simulink model "BattEv_Simscape"  (R2023b)
settings: Solver=ode23t  StartTime=0  StopTime=inf  RelTol=1e-3  EnableMultiTasking=on
model workspace (MAT data in the model file):
  Active_Scenario_Index = 1
  BattCurrent = [0 0.1 0.2 0.3 0.4 0.5 0.6 0.7 0.8 0.9 1 1.1 ... (49482 elements, 24741x2)]
  BattSocInit = 0.75
  BattTempInit = 25
  Battery.SOC_LUT = [0.01 0.02 0.03 0.04 0.05 0.06 0.07 0.08 0.09 0.1 0.11 0.12 0.13 0.14 0.15 0.16 0.17 0.18 0.19 0.2 0.21 0.22 0.23 0.24 0.25 0.26 0.27 0.28 0.29 0.3 0.31 0.32 0.33 0.34 0.35 0.36 0.37 0.38 0.39 0.4 0.41 0.42 0.43 0.44 0.45 0.46 0.47 0.48 0.49 0.5 0.51 0.52 0.53 0.54 0.55 0.56 0.57 0.58 0.59 0.6 0.61 0.62 0.63 0.64 0.65 0.66 0.67 0.68 0.69 0.7 0.71 0.72 0.73 0.74 0.75 0.76 0.77 0.78 0.79 0.8 0.81 0.82 0.83 0.84 0.85 0.86 0.87 0.88 0.89 0.9 0.91 0.92 0.93 0.94 0.95 0.96 0.97 0.98 0.99 1]
  Battery.Temperature_LUT = [-10 0 25 40]
  Battery.Capacity_LUT = [4.04528301887 4.19622641509 4.8 4.73962264151]
  Battery.Em_LUT = [2.67308083891 2.74411674384 2.80408613071 2.86247711994 2.90851059763 2.94904306488 2.9829846776 3.01467102589 3.04031502638 3.06256828113 3.08180972392 3.09994219643 ... (400 elements, 100x4)]
  Battery.R0_LUT = [0.0569026752707 0.0575506938969 0.0576730924021 0.0575627404981 0.0573787336615 0.0571931123197 0.0568199985482 0.056411926464 0.0561974340667 0.0560805640861 0.0557640899305 0.055275807865 ... (400 elements, 100x4)]
  Battery.R1_LUT = [0.0035 0.0035 0.0035 0.0035 0.0035 0.0035 0.0035 0.0035 0.0035 0.0035 0.0035 0.0035 ... (400 elements, 100x4)]
  Battery.C1_LUT = [5000 5000 5000 5000 5000 5000 5000 5000 5000 5000 5000 5000 ... (400 elements, 100x4)]
  Battery.Mass = 0.047
  Battery.ThermalMass = 44
  Battery.R_bleed = 20
  Battery.h_conv = 5
  Battery.cell_area = 0.0037
  Battery.TempInit = 25
  Battery.SOCInit = 0.75
  Battery.Model = 'panasonic ncr18650bd'
  Battery.DischargeCycle_LUT = [1 5 9 13 17 21 25 29 33 37 41 45 49 53 57 61 65 69 73 77 81 85 89 93 97 101 105 109 113 117 121 125 129 133 137 141 145 149 153 157 161 165 169 173 177 181 185 189 193 197 201 205 209 213 217 221 225 229 233 237 241 245 249 253 257 261 265 269 273 277 281 285 289 293 297 301 305 309 313 317]
  Battery.deltaEm_LUT = [0 -0.363115641304 -0.600096647258 -0.689070000839 -0.76773380251 -0.846397604181 -0.926368385458 -0.992711297521 -1.05704974111 -1.12227693902 -1.19018070587 -1.25808447272 -1.31699459748 -1.35876443799 -1.40168267642 -1.44460091485 -1.48751915327 -1.5304373917 -1.57335563013 -1.62198241593 -1.67232184498 -1.71858340023 -1.76179802551 -1.8050126508 -1.84822727608 -1.8917937136 -1.93575272784 -1.97971174208 -2.02367075632 -2.06762977056 -2.11171979109 -2.15588700406 -2.19980020032 -2.24365853098 -2.28751686164 -2.33137519231 -2.37523352297 -2.41909185363 -2.45982559031 -2.49599372373 -2.53216185715 -2.56832999058 -2.604498124 -2.64066625743 -2.67683439085 -2.71300252428 -2.7491706577 -2.78367585394 -2.81632179346 -2.8483348579 -2.88034792233 -2.91236098677 -2.94437405121 -2.97638711564 -3.00840018008 -3.04041324451 -3.07260346059 -3.10359008254 -3.13082308991 -3.15805609728 -3.18528910464 -3.21252211201 -3.23975511938 -3.26698812675 -3.29422113412 -3.32122400938 -3.3463475604 -3.37152613073 -3.39670470105 -3.42188327138 -3.4470618417 -3.47224041203 -3.49938358795 -3.52900276724 -3.55862194653 -3.58824112582 -3.6178603051 -3.64748858268 -3.67711690909 -3.70674523549]
  Battery.deltaCapacity_LUT = [0 -0.860019120059 -1.71332421702 -2.0819400264 -2.45055583577 -2.81917164515 -3.18778745452 -3.48884924257 -3.7808148236 -4.07278040463 -4.36474598566 -4.6567115667 -4.91000721732 -5.08494410056 -5.2598809838 -5.43481786703 -5.60975475027 -5.78469163351 -5.95962851674 -6.13456539998 -6.30950228322 -6.47026795816 -6.62044510558 -6.77062225299 -6.92079940041 -7.07097654783 -7.22115369524 -7.37133084266 -7.52150799007 -7.67168513749 -7.82230984162 -7.97319825819 -8.12408667477 -8.27497509134 -8.42586350792 -8.57675192449 -8.72764034107 -8.87852875764 -9.01789522921 -9.13717923376 -9.25646323831 -9.37574724285 -9.4950312474 -9.61431525195 -9.73359925649 -9.85288326104 -9.97216726558 -10.0914512701 -10.2059878191 -10.3183039593 -10.4306200996 -10.5429362398 -10.65525238 -10.7675685203 -10.8798846605 -10.9922008008 -11.104516941 -11.2125891929 -11.3075699376 -11.4025506823 -11.4975314271 -11.5925121718 -11.6874929166 -11.7824736613 -11.877454406 -11.9716325175 -12.0588579537 -12.1460833899 -12.2333088261 -12.3205342623 -12.4077596986 -12.4949851348 -12.5890165008 -12.6916254178 -12.7942343349 -12.8968432519 -12.999452169 -13.102061086 -13.2046700031 -13.3072789201]
  Battery.cond_thickness = 0.001
  Battery.thermal_conductivity = 205
  CellType = 1
  EV_current = 200
  EV_motion = [20 4 0.8]
  EV_sf = 2000
  Fs = 0
  Fv = 0.0025
  Jcomp = 0.0227
  Ki = 251.3274
  Kisa = 346.6583
  Kp_d = 0.47149
  Kp_q = 0.52125
  Ksa = 85.4316
  Ksf = 1996.2651
  Ld = 0.0003752
  Ldq = [0.0003752 0.0004148]
  Lq = 0.0004148
  Mechanical = [0.0227 0.0025 0]
  Np_Module = 31
  Ns_Module = 24
  NumModules = 4
  OverCellVoltageLimit = 4.19999980927
  P = 4
  PolePairs = 4
  R_bleed = 20
  Rs = 0.2
  T_eff_bp = [0 32.1428571429 64.2857142857 96.4285714286 128.571428571 160.714285714 192.857142857 225 257.142857143 289.285714286 321.428571429 353.571428571 385.714285714 417.857142857 450]
  T_env = 30
  T_init = 303.15
  T_max = 450
  T_mtpa = [0 13.3131834767 26.6278836885 39.9456159322 53.2678926341 66.5962219318 79.9321062746 93.277041051 106.632513247 120.000000141]
  T_set = 20.5
  Tc = 0.02
  TempInit = 288.15
  TestCase = 1
  UnderCellVoltageLimit = 2.5
  ba = 3.4029
  cell_area = 0.101908
  efficiency_table = [86.7  86.7  86.7  86.7  86.7  86.7  86.7  86.7  86.7  86.7  86.7  86.7  86.7  86.7  86.7; 86.7  86.7  86.7  86.7  86.7  86.7  86.7  86.7  86.7  86.7  86.7  86.7  86.7  86.7  86.7; 86.7  86.7  91.8  91.8  91.8  91.8  91.8  91.8  91.8  91.8  89.76  89.76  89.76  89.76  89.76; 86.7  86.7  93.84  93.84  93.84  93.84  93.84  93.84  93.84  93.84  93.84  91.8  91.8  91.8  91.8; 86.7  86.7  93.84  93.84  94.86  94.86  94.86  94.86  93.84  93.84  93.84  91.8  91.8  91.8  91.8; 86.7  86.7  94.86  95.88  95.88  95.88  95.88  95.88  95.88  95.88  95.88  95.88  95.88  95.88  95.88; 86.7  86.7  94.86  95.88  95.88  96.9  96.9  96.9  96.9  96.9  96.9  96.9  96.9  96.9  96.9; 86.7  86.7  94.86  95.88  95.88  96.9  96.9  96.9  96.9  96.9  96.9  96.9  96.9  96.9  96.9; 86.7  86.7  94.86  95.88  96.9  96.9  96.9  96.9  96.9  96.9  96.9  96.9  96.9  96.9  96.9; 86.7  86.7  94.86  95.88  96.9  96.9  96.9  96.9  96.9  96.9  96.9  96.9  96.9  96.9  96.9; 86.7  86.7  94.86  95.88  95.88  95.88  95.88  95.88  95.88  95.88  95.88  95.88  95.88  95.88  95.88; 86.7  86.7  91.8  93.84  94.86  94.86  94.86  94.86  94.86  94.86  94.86  94.86  94.86  94.86  94.86]
  h_conv = 5
  id_mtpa = [0 -0.114523352646 -0.457989076459 -1.03008464374 -1.83029075221 -2.85788367342 -4.11193850568 -5.59133329791 -7.29475400168 -9.22070020138]
  idq0 = [0 0]
  idq_limits = [-9.220699542 166.993501392 167.247872355]
  iq_mtpa = [0 18.5827440345 37.1633719111 55.7397734896 74.3098506185 92.871523015 111.422734008 129.961456105 148.485696337 166.993501356]
  lambda_pm = 0.1194
  losses_table = [0  0  0  0  0  0  0  0  0  0  0  0  0  0  0; 0  0  0  0  0  0  0  0  0  0  0  0  0  0  0; 0  0  0  0  0  0  0  0  0  0  0  0  0  0  0; 0  0  0  0  0  0  0  0  0  0  0  0  0  0  0; 0  0  0  0  0  0  0  0  0  0  0  0  0  0  0; 0  0  0  0  0  0  0  0  0  0  0  0  0  0  0; 0  0  0  0  0  0  0  0  0  0  0  0  0  0  0; 0  0  0  0  0  0  0  0  0  0  0  0  0  0  0; 0  0  0  0  0  0  0  0  0  0  0  0  0  0  0; 0  0  0  0  0  0  0  0  0  0  0  0  0  0  0; 0  0  0  0  0  0  0  0  0  0  0  0  0  0  0; 0  0  0  0  0  0  0  0  0  0  0  0  0  0  0]
  mdot_rev = 0.01
  mechanical = [0.0227 0.0025 0]
  omega_init = 0
  pipe.length = 75
  pipe.Dh = 2.5
  pipe.area = 4.90873852123
  power_max = 211000
  pump.omega = 4000
  pump.displacement = 40
  radiator.area_air = 0.15
  radiator.volume_air = 0.01
  radiator.area_liquid = 0.000314159265359
  radiator.volume_liquid = 0.000157079632679
  radiator.mdot_air = [0.1 8]
  radiator.mdot_liquid = [0.1 5]
  radiator.SD = [1  9; 2  10]
  radiator.dp_air = [0.003 0.01]
  radiator.dp_liquid = [0.005 0.02]
  t_sim = 2474
  tank.volume = 10
  tank.area = 0.0625
  tank.area_wall = 0.375
  theta_init = 0
  torque_max = 450
  ts = 0.1
  valve.area = 4.90873852123
  valve.opening = 4.81056375081
  valve.area_leak = 1e-05
  w_eff_bp = [0 1600 3200 4477.56 4800 6400 8000 9600 11200 12800 14400 16000]
libraries: autolibpowerinfoutils x10, fl_lib x7, nesl_utility_internal x6, ee_lib x1
(part 1 of 2)
settings Model: DataDictionary=DD_Battery.sldd  ModifiedByFormat=The MathWorks, Inc.  SimulationMode=accelerator  Creator=The MathWorks, Inc.  LastModifiedBy=The MathWorks, Inc.
settings SolverCC: SolverJacobianMethodControl=FullPerturbation  ZeroCrossAlgorithm=Adaptive  AlgebraicLoopSolver=TrustRegion  AutoInsertRateTranBlk=on  DecoupledContinuousIntegration=on  MinimalZcImpactIntegration=on  MaxZcPerStep=1
settings DataIOCC: SaveOutput=off  DSMLogging=off  SaveTime=off  ReturnWorkspaceOutputs=off
settings OptimizationCC: ReuseModelBlockBuffer=off
settings DebuggingCC: ArtificialAlgebraicLoopMsg=none  UnderspecifiedInitializationDetection=Classic  MergeDetectMultiDrivingBlocksExec=none  IgnoredZcDiagnostic=none  UnconnectedInputMsg=warning  UnconnectedOutputMsg=warning  UnconnectedLineMsg=warning  ModelReferenceExtraNoncontSigs=none  PregeneratedLibrarySubsystemCodeDiagnostic=none  SubsystemReferenceDiagnosticForUnitTest=warning  ArithmeticOperatorsInVariantConditions=warning
settings ModelReferenceCC: UpdateModelReferenceTargets=IfOutOfDate  EnableRefExpFcnMdlSchedulingChecks=on  ModelReferenceMinAlgLoopOccurrences=on  PropagateSignalLabelsOutOfModel=off
settings SFSimCC: SimUseLocalCustomCode=off
settings RTWCC: RTWUseLocalCustomCode=off  DLArmComputeVersion=19.05
settings CodeAppCC: StateflowObjectComments=on
settings GRTTargetCC: TargetLangStandard=C89/C90 (ANSI)
settings ConfigComp: CovMetricSettings=dsw  CovSaveCumulativeToWorkspaceVar=on  CovSaveSingleToWorkspaceVar=on  CovExternalEMLEnable=off
settings SimscapeCC: SimscapeLogSimulationStatistics=on  SimscapeLogToSDI=on  SimscapeLogOpenViewer=on  SimscapeLogLimitData=off

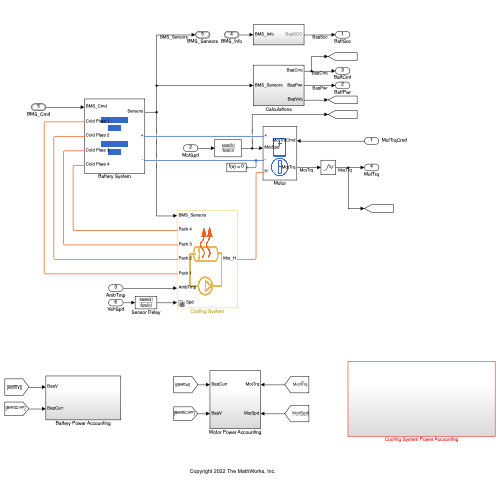
[thumbnail: Simulink's stored preview of the top-level diagram]
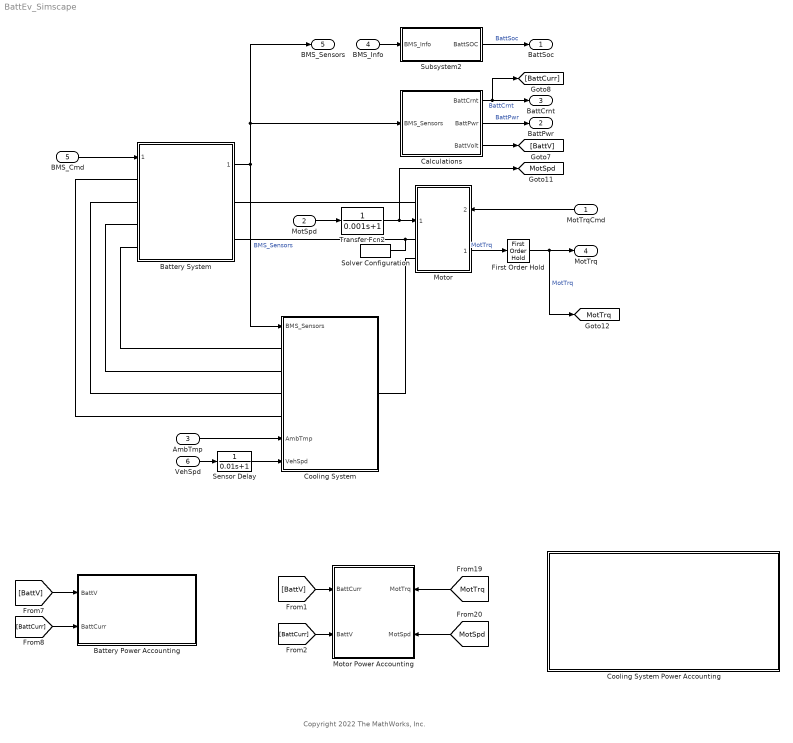
== system BattEv_Simscape ==
  note: Copyright 2022 The MathWorks, Inc.
  MotTrqCmd : Inport
  MotSpd : Inport  Port=2
  AmbTmp : Inport  Port=3
  BMS_Info : Inport  Port=4  OutDataTypeStr=Bus: BMS_Info
  BMS_Cmd : Inport  Port=5  OutDataTypeStr=Bus: BMS_Cmd
  VehSpd : Inport  Port=6
  Battery Power Accounting : Subsystem
  Battery System : Subsystem  ReferencedSubsystem=Battery_Model
  Calculations : Subsystem
  Cooling System : Subsystem  Variant=on  VariantControlMode=label  VariantControl=Choice  LabelModeActiveChoice=1
      settings: PortSchema="{\"entries\":[{\"content\":{\"sides\":[{\"content\":{\"connectorIds\":[\"In1\",\"LConn1\",\"LConn2\",\"LConn3\",\"LConn4\",\"In2\",\"In3\"]},\"type\":\"ConnectorPlacement.EquallySpacedRectSide\",\"uuid\":\"c167541e-e4b9-49e2-9aa7-1fe3e992d52d\"},{\"content\":{\"connectorIds\":[\"RConn1\"],\"side\":\"RIGHT\"},\"type\":\"ConnectorPlacement.EquallySpacedRectSide\",\"uuid\":\"bae8285f-2b84-4cb8-84af-359175be4c5c\"},{\"content\":{\"connectorIds\":[],\"side\":\"TOP\"},\"type\":\"ConnectorPlacement.EquallySpacedRectSide\",\"uuid\":\"a9a12dc9-88d6-4e34-9217-c23bb475a40a\"}]},\"type\":\"ConnectorPlacement.EquallySpacedConnector\",\"uuid\":\"22e6fce0-8f6d-4e5f-a37f-94d98424337f\"}],\"packageUris\":[\"http://schema.mathworks.com/mf0/Connector/R2020b\"],\"version\":\"1.0\"}"
  Cooling System Power Accounting : Subsystem
  First Order Hold : FirstOrderHold  ErrorTolerance=inf  AllowContinuousInput=on
  Motor : Subsystem
      settings: PortSchema="{\"entries\":[{\"content\":{\"sides\":[{\"content\":{\"connectorIds\":[\"LConn1\",\"In1\",\"LConn2\",\"LConn3\"]},\"type\":\"ConnectorPlacement.EquallySpacedRectSide\",\"uuid\":\"9597c387-ee3f-4b24-bb5e-e93595cd0799\"},{\"content\":{\"connectorIds\":[\"In2\",\"Out1\"],\"side\":\"RIGHT\"},\"type\":\"ConnectorPlacement.EquallySpacedRectSide\",\"uuid\":\"f263f5bf-92e3-41e6-b8e0-90892aa1ca09\"},{\"content\":{\"connectorIds\":[],\"side\":\"TOP\"},\"type\":\"ConnectorPlacement.EquallySpacedRectSide\",\"uuid\":\"fc14820c-8222-4fb0-a838-a8d38af04827\"}]},\"type\":\"ConnectorPlacement.EquallySpacedConnector\",\"uuid\":\"4528e8dd-d5c0-4035-a357-37b593191d34\"}],\"packageUris\":[\"http://schema.mathworks.com/mf0/Connector/R2020b\"],\"version\":\"1.0\"}"
      mask Display: image('emotor_simplified_IMAGE.png'); % Use "Edit Image" on toolstrip to change.
  Motor Power Accounting : Subsystem
      settings: PortSchema="{\"entries\":[{\"content\":{\"sides\":[{\"content\":{\"connectorIds\":[\"In1\",\"In2\"]},\"type\":\"ConnectorPlacement.EquallySpacedRectSide\",\"uuid\":\"6ec4812d-f6a8-428e-ab71-0e64a82e557b\"},{\"content\":{\"connectorIds\":[\"In3\",\"In4\"],\"side\":\"RIGHT\"},\"type\":\"ConnectorPlacement.EquallySpacedRectSide\",\"uuid\":\"a1192fa4-ef5f-453a-86cc-222a9b7953b2\"},{\"content\":{\"connectorIds\":[],\"side\":\"TOP\"},\"type\":\"ConnectorPlacement.EquallySpacedRectSide\",\"uuid\":\"391d63f3-8abc-4151-8569-a2196654f909\"}]},\"type\":\"ConnectorPlacement.EquallySpacedConnector\",\"uuid\":\"660d9ac6-f464-40a8-9602-452be741244a\"}],\"packageUris\":[\"http://schema.mathworks.com/mf0/Connector/R2020b\"],\"version\":\"1.0\"}"
  Sensor Delay : TransferFcn  Denominator=[0.01 1]
  Solver Configuration : nesl_utility_internal/Solver Configuration  PhysicalDomain=network_engine_domain  SubClassName=solver  LeftPortType=input  RightPortType=generic  Tones=[]  Harmonics=[]  SimulateNoise=off  Profile=off  UseLocalSampling=off  EnableSwitchedLinearOptims=on  FrequencyDomain=off  UseCCode=off  RelTol=0.001  AbsTol=1e-06  MinStep=1e-09  ToWorkspace=off  RevertToSquareIcSolve=off  NumHomotopyIterations=100  PhasorMode=off  PhasorModeNumHarmonics=1  ConsistencySolver=NEWTON_FTOL  IndexReductionMethod=DerivativeReplacement  DoDC=off  ResidualTolerance=1e-09  ConsistencyTolSource=GLOBAL  ConsistencyAbsTol=0.001  ConsistencyRelTol=0.001  ConsistencyTolFactor=0.001  UseLocalSolver=on  LocalSolverChoice=NE_BACKWARD_EULER_ADVANCER  ResolveIndetEquations=on  FunctionEvalNumThread=1  LocalSolverSampleTime=ts  DoFixedCost=on  MaxNonlinIter=3  MaxModeIter=2  ComputeImpulses=off  ImpulseIterations=2  LinearAlgebra=auto  LinearAlgebraNumThread=0  EquationFormulation=NE_TIME_EF  DelaysMemoryBudget=1024  AutomaticFiltering=off  FilteringTimeConstant=0.001  PartitionStorageMethod=AS_NEEDED  PartitionMemoryBudget=1024  PartitionMethod=FAST  MultibodyUseLocalSolver=off  MultibodyLocalSolverChoice=ODE1  MultibodyLocalSolverSampleTime=0.001
  Subsystem2 : Subsystem
  Transfer Fcn2 : TransferFcn  Denominator=[0.001 1]
  BattSoc : Outport  VectorParamsAs1DForOutWhenUnconnected=off
  BattPwr : Outport  Port=2  VectorParamsAs1DForOutWhenUnconnected=off
  BattCrnt : Outport  Port=3  VectorParamsAs1DForOutWhenUnconnected=off
  MotTrq : Outport  Port=4  VectorParamsAs1DForOutWhenUnconnected=off
  BMS_Sensors : Outport  Port=5  OutDataTypeStr=Bus: Sensors  VectorParamsAs1DForOutWhenUnconnected=off  BusOutputAsStruct=on
  tag scope: MotSpd=global, MotTrq=global
  wires:
  BMS_Cmd/1 -> Battery System/1
  Subsystem2/1(BattSOC) -> BattSoc/1  "BattSoc"
  MotSpd/1 -> Transfer Fcn2/1
  AmbTmp/1 -> Cooling System/2(AmbTmp)
  Calculations/1(BattCrnt) -> BattCrnt/1, [BattCurr]  "BattCrnt"
  VehSpd/1 -> Sensor Delay/1
  Battery System/1 -> BMS_Sensors/1, Calculations/1(BMS_Sensors), Cooling System/1(BMS_Sensors)  "BMS_Sensors"
  Sensor Delay/1 -> Cooling System/3(VehSpd)
  BMS_Info/1 -> Subsystem2/1(BMS_Info)
  Motor/1(MotTrq) -> First Order Hold/1  "MotTrq"
  Calculations/3(BattVolt) -> [BattV]
  Calculations/2(BattPwr) -> BattPwr/1  "BattPwr"
  MotTrqCmd/1 -> Motor/2(MotTrqCmd)
  [MotTrq] -> Motor Power Accounting/3(MotTrq)
  [BattV] -> Motor Power Accounting/1(BattCurr)
  [BattCurr] -> Battery Power Accounting/2(BattCurr)
  [MotSpd] -> Motor Power Accounting/4(MotSpd)
  [BattCurr] -> Motor Power Accounting/2(BattV)
  [BattV] -> Battery Power Accounting/1(BattV)
  First Order Hold/1 -> [MotTrq], MotTrq/1  "MotTrq"
  Transfer Fcn2/1 -> [MotSpd], Motor/1(MotSpd)
  connections:
  Motor/LConn2 -- Battery System/RConn2 -- Solver Configuration/RConn1
  Battery System/RConn1 -- Motor/LConn1
  Cooling System/LConn4 -- Battery System/LConn1
  Cooling System/LConn3 -- Battery System/LConn2
  Cooling System/LConn2 -- Battery System/LConn3
  Cooling System/LConn1 -- Battery System/LConn4
  Motor/LConn3 -- Cooling System/RConn1
